simulink model "Cascaded_H_Bridge_Inverter"  (R2017a)
settings: Solver=VariableStepAuto  StartTime=0.0  StopTime=20e-3  MaxStep=1e-4  RelTol=1e-3
values from neighbouring files (symbols this model uses):
  Fs = 10000    [sequence_generator.m]
  o11 = zeros(1, Fs)    [sequence_generator.m]
  o13 = zeros(1, Fs)    [sequence_generator.m]
  o21 = zeros(1, Fs)    [sequence_generator.m]
  o23 = zeros(1, Fs)    [sequence_generator.m]
  p = 20e-3    (= 0.02)    [sequence_generator.m]
libraries: powerlib_meascontrol x37, powerlib x26, simulink x8
settings Model: Creator=Abubakar  LastModifiedBy=Abubakar

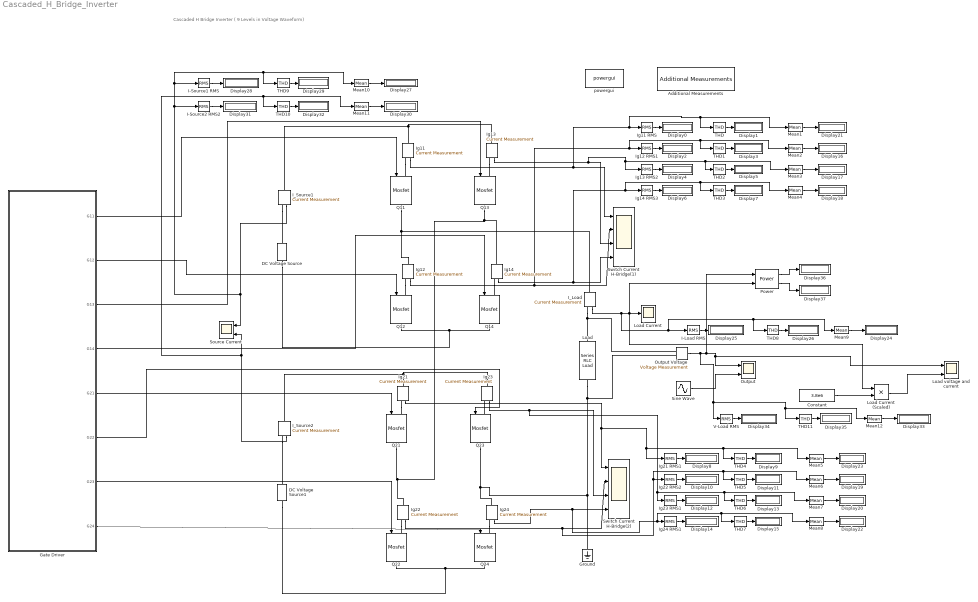
== system Cascaded_H_Bridge_Inverter ==
  note: Cascaded H Bridge Inverter
      | ( 9 Levels in Voltage Waveform)
  Additional Measurements : powerlib/Measurements/Additional Measurements  SystemSampleTime=-1
      settings: SourceProductName=Simscape Power Systems  SourceProductBaseCode=PS
  Constant : Constant  Value=3.8e6
  DC Voltage Source : powerlib/Electrical Sources/DC Voltage Source  Amplitude=10000  Measurements=None
  DC Voltage Source1 : powerlib/Electrical Sources/DC Voltage Source  Amplitude=30000  Measurements=None
  Display{0..37} (38 alike) : Display
  Gate Driver : Subsystem
  Ground : powerlib/Elements/Ground  LConnTagsString=a
  I-Load RMS : powerlib_meascontrol/Measurements/RMS  TrueRMS=on  Freq=50  RMSInit=0  Ts=0
  I-Source1 RMS : powerlib_meascontrol/Measurements/RMS  TrueRMS=on  Freq=50  RMSInit=0  Ts=0
  I-Source2 RMS2 : powerlib_meascontrol/Measurements/RMS  TrueRMS=on  Freq=50  RMSInit=0  Ts=0
  I_Load : powerlib/Measurements/Current Measurement  PhasorSimulation=off  OutputType=Complex  PSBequivalent=0
  I_Source1 : powerlib/Measurements/Current Measurement  PhasorSimulation=off  OutputType=Complex  PSBequivalent=0
  I_Source2 : powerlib/Measurements/Current Measurement  PhasorSimulation=off  OutputType=Complex  PSBequivalent=0
  Ig{11..14,21..24} (8 alike) : powerlib/Measurements/Current Measurement  PhasorSimulation=off  OutputType=Complex  PSBequivalent=0
  Ig11 RMS : powerlib_meascontrol/Measurements/RMS  TrueRMS=on  Freq=50  RMSInit=0  Ts=0
  Ig12 RMS1 : powerlib_meascontrol/Measurements/RMS  TrueRMS=on  Freq=50  RMSInit=0  Ts=0
  Ig13 RMS2 : powerlib_meascontrol/Measurements/RMS  TrueRMS=on  Freq=50  RMSInit=0  Ts=0
  Ig14 RMS3 : powerlib_meascontrol/Measurements/RMS  TrueRMS=on  Freq=50  RMSInit=0  Ts=0
  Ig21 RMS1 : powerlib_meascontrol/Measurements/RMS  TrueRMS=on  Freq=50  RMSInit=0  Ts=0
  Ig22 RMS2 : powerlib_meascontrol/Measurements/RMS  TrueRMS=on  Freq=50  RMSInit=0  Ts=0
  Ig23 RMS1 : powerlib_meascontrol/Measurements/RMS  TrueRMS=on  Freq=50  RMSInit=0  Ts=0
  Ig24 RMS1 : powerlib_meascontrol/Measurements/RMS  TrueRMS=on  Freq=50  RMSInit=0  Ts=0
  Load : powerlib/Elements/Series RLC Load  LConnTagsString=a  RConnTagsString=__new0  NominalVoltage=2.5e4  NominalFrequency=50  ActivePower=100  InductivePower=0  CapacitivePower=0  Setx0=off  InitialVoltage=0  SetiL0=off  InitialCurrent=0  Measurements=None  LoadType=constant PQ
  Load Current : Scope
  Load Current (Scaled) : Product
  Load voltage and current : Scope  NumInputPorts=2
  Mean{1..12} (12 alike) : powerlib_meascontrol/Measurements/Mean  Freq=60  Vinit=0  Ts=0
  Output : Scope  NumInputPorts=2
  Output Voltage : powerlib/Measurements/Voltage Measurement  PhasorSimulation=off  OutputType=Complex  PSBequivalent=0
  Power : powerlib_meascontrol/Measurements/Power  Freq=50  Vinit=[1, 0]  Iinit=[1, 0]  Ts=0
      settings: SourceProductName=Simscape Power Systems
  Q{11..14,21..24} (8 alike) : powerlib/Power Electronics/Mosfet  Ron=0.0001  Lon=0  Rd=0.0001  Vfd=0  IC=0  Rs=1e5  Cs=inf  Measurements=off
  Sine Wave : Sin  Amplitude=40000  Frequency=2*pi*(1/p)  SampleTime=0
  Source Current : Scope  NumInputPorts=2
  Switch Current H-Bridge(1) : Scope  NumInputPorts=4
  Switch Current H-Bridge(2) : Scope  NumInputPorts=4
  THD{,1..11} (12 alike) : powerlib_meascontrol/Measurements/THD  Freq=50  Ts=0
  V-Load RMS : powerlib_meascontrol/Measurements/RMS  TrueRMS=on  Freq=50  RMSInit=0  Ts=0
  powergui : powerlib/powergui  Priority=1  SimulationMode=Continuous  SampleTime=50e-6  frequency=60  Iterations=50  frequencyindice=0  Pbase=100e6  ErrMax=1e-4  UnitsV=kV  UnitsW=MW  buscounter=0  FunctionMessages=off  echomessages=off  EnableUseOfTLC=off  CurrentSourceSwitches=off  DisableSnubberDevices=off  DisableRonSwitches=off  DisableVfSwitches=off  DisplayEquations=off  SolverType=Tustin/Backward Euler (TBE)  Interpol=off  ExternalGateDelay=off  methode=off  Ts=100  x0status=blocks  SPID=on  SwTol=0  HookPort=off  RestoreLinks=warning  ResistiveCurrentMeasurement=off  Frange=[0:2:500]  Ylog=off  Xlog=on  ShowGrid=off  save=off  variable=ZData  structure=OutputData  ZoomFFT=off  StartTime=0  cycles=2  DisplayStyle=1  fundamental=50  FreqAxis=on  MaxFrequency=1000  frequencyindicesteady=1  RmsSteady=1  display=off
  wires:
  Gate Driver/1(G11) -> Q11/1
  Gate Driver/2(G12) -> Q12/1
  Gate Driver/3(G13) -> Q13/1
  Gate Driver/4(G14) -> Q14/1
  Gate Driver/5(G21) -> Q21/1
  Gate Driver/6(G22) -> Q23/1
  Gate Driver/7(G23) -> Q22/1
  Gate Driver/8(G24) -> Q24/1
  Sine Wave/1 -> Output/2
  Ig11/1 -> Mean1/1, THD/1, Ig11 RMS/1, Switch Current H-Bridge(1)/1
  Ig12/1 -> Mean2/1, THD1/1, Ig12 RMS1/1, Switch Current H-Bridge(1)/2
  Ig13/1 -> Mean3/1, THD2/1, Ig13 RMS2/1, Switch Current H-Bridge(1)/3
  Ig14/1 -> Mean4/1, THD3/1, Ig14 RMS3/1, Switch Current H-Bridge(1)/4
  Ig21/1 -> Mean5/1, THD4/1, Ig21 RMS1/1, Switch Current H-Bridge(2)/1
  Ig22/1 -> Mean6/1, THD5/1, Ig22 RMS2/1, Switch Current H-Bridge(2)/2
  Ig23/1 -> Mean7/1, THD6/1, Ig23 RMS1/1, Switch Current H-Bridge(2)/3
  Ig24/1 -> Mean8/1, THD7/1, Ig24 RMS1/1, Switch Current H-Bridge(2)/4
  THD/1 -> Display1/1
  Ig11 RMS/1 -> Display0/1
  Ig12 RMS1/1 -> Display2/1
  THD1/1 -> Display3/1
  THD2/1 -> Display5/1
  Ig13 RMS2/1 -> Display4/1
  Ig14 RMS3/1 -> Display6/1
  THD3/1 -> Display7/1
  THD7/1 -> Display15/1
  Ig24 RMS1/1 -> Display14/1
  Ig23 RMS1/1 -> Display12/1
  THD6/1 -> Display13/1
  THD5/1 -> Display11/1
  Ig22 RMS2/1 -> Display10/1
  Ig21 RMS1/1 -> Display8/1
  THD4/1 -> Display9/1
  Mean1/1 -> Display21/1
  Mean2/1 -> Display16/1
  Mean3/1 -> Display17/1
  Mean4/1 -> Display18/1
  Mean8/1 -> Display22/1
  Mean7/1 -> Display20/1
  Mean6/1 -> Display19/1
  Mean5/1 -> Display23/1
  Mean9/1 -> Display24/1
  THD8/1 -> Display26/1
  I-Load RMS/1 -> Display25/1
  I_Load/1 -> Mean9/1, THD8/1, I-Load RMS/1, Load Current (Scaled)/1, Power/2, Load Current/1
  I_Source1/1 -> I-Source2 RMS2/1, I-Source1 RMS/1, THD9/1, Mean10/1, Source Current/1
  I-Source1 RMS/1 -> Display28/1
  THD9/1 -> Display29/1
  Mean10/1 -> Display27/1
  Mean11/1 -> Display30/1
  THD10/1 -> Display32/1
  I-Source2 RMS2/1 -> Display31/1
  I_Source2/1 -> Mean11/1, THD10/1, Source Current/2
  Output Voltage/1 -> THD11/1, Mean12/1, V-Load RMS/1, Power/1, Load voltage and current/1, Output/1
  V-Load RMS/1 -> Display34/1
  THD11/1 -> Display35/1
  Mean12/1 -> Display33/1
  Power/1 -> Display36/1
  Power/2 -> Display37/1
  Load Current (Scaled)/1 -> Load voltage and current/2
  Constant/1 -> Load Current (Scaled)/2
  connections:
  Ig13/LConn1 -- I_Source1/LConn1 -- Ig11/LConn1
  Q11/RConn1 -- I_Load/LConn1 -- Ig12/LConn1
  Q12/RConn1 -- DC Voltage Source/LConn1 -- Q14/RConn1
  Ig21/LConn1 -- I_Source2/LConn1 -- Ig23/LConn1
  Q22/RConn1 -- DC Voltage Source1/LConn1 -- Q24/RConn1
  Q13/RConn1 -- Ig22/LConn1 -- Q21/RConn1 -- Ig14/LConn1
  Q23/RConn1 -- Ig24/LConn1 -- Load/RConn1 -- Output Voltage/LConn2 -- Ground/LConn1
  Ig11/RConn1 -- Q11/LConn1
  Ig13/RConn1 -- Q13/LConn1
  Ig12/RConn1 -- Q12/LConn1
  Ig14/RConn1 -- Q14/LConn1
  Ig23/RConn1 -- Q23/LConn1
  Ig21/RConn1 -- Q21/LConn1
  Ig24/RConn1 -- Q24/LConn1
  Ig22/RConn1 -- Q22/LConn1
  Output Voltage/LConn1 -- I_Load/RConn1 -- Load/LConn1
  I_Source1/RConn1 -- DC Voltage Source/RConn1
  I_Source2/RConn1 -- DC Voltage Source1/RConn1

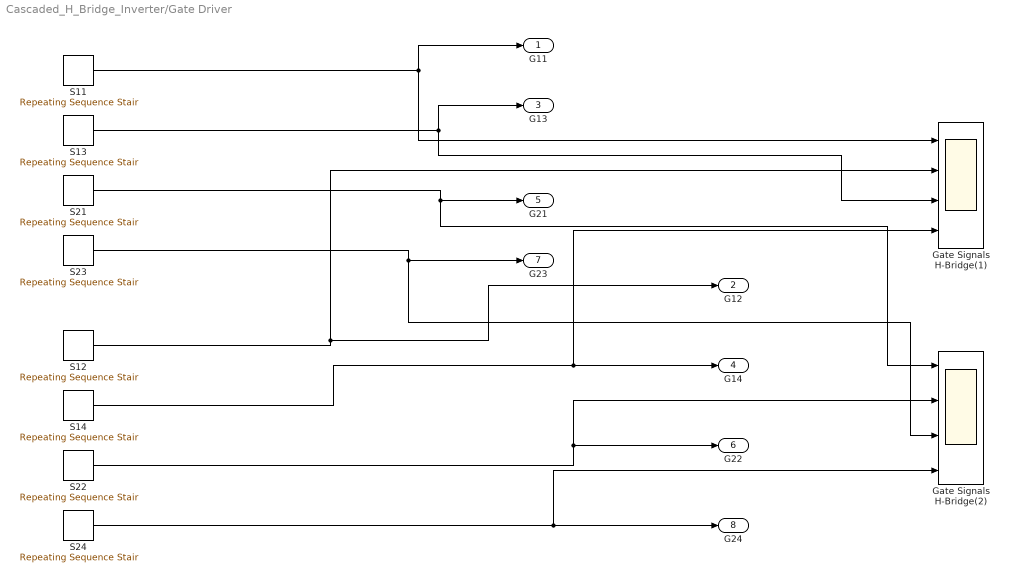
== system Cascaded_H_Bridge_Inverter/Gate Driver ==
  Gate Signals H-Bridge(1) : Scope  NumInputPorts=4
  Gate Signals H-Bridge(2) : Scope  NumInputPorts=4
  S11 : simulink/Sources/Repeating Sequence Stair  OutValues=o11'  tsamp=(p/Fs)  OutMin=[]  OutMax=[]  OutDataTypeStr=double  OutputDataTypeScalingMode=double  OutDataType=fixdt(0,8)  ConRadixGroup=Best Precision: Vector-wise  OutScaling=2^-12
  S12 : simulink/Sources/Repeating Sequence Stair  OutValues=~o11'  tsamp=(p/Fs)  OutMin=[]  OutMax=[]  OutDataTypeStr=double  OutputDataTypeScalingMode=double  OutDataType=fixdt(0,8)  ConRadixGroup=Best Precision: Vector-wise  OutScaling=2^-12
  S13 : simulink/Sources/Repeating Sequence Stair  OutValues=o13'  tsamp=(p/Fs)  OutMin=[]  OutMax=[]  OutDataTypeStr=double  OutputDataTypeScalingMode=double  OutDataType=fixdt(0,8)  ConRadixGroup=Best Precision: Vector-wise  OutScaling=2^-12
  S14 : simulink/Sources/Repeating Sequence Stair  OutValues=~o13'  tsamp=(p/Fs)  OutMin=[]  OutMax=[]  OutDataTypeStr=double  OutputDataTypeScalingMode=double  OutDataType=fixdt(0,8)  ConRadixGroup=Best Precision: Vector-wise  OutScaling=2^-12
  S21 : simulink/Sources/Repeating Sequence Stair  OutValues=o21'  tsamp=(p/Fs)  OutMin=[]  OutMax=[]  OutDataTypeStr=double  OutputDataTypeScalingMode=double  OutDataType=fixdt(0,8)  ConRadixGroup=Best Precision: Vector-wise  OutScaling=2^-12
  S22 : simulink/Sources/Repeating Sequence Stair  OutValues=~o21'  tsamp=(p/Fs)  OutMin=[]  OutMax=[]  OutDataTypeStr=double  OutputDataTypeScalingMode=double  OutDataType=fixdt(0,8)  ConRadixGroup=Best Precision: Vector-wise  OutScaling=2^-12
  S23 : simulink/Sources/Repeating Sequence Stair  OutValues=o23'  tsamp=(p/Fs)  OutMin=[]  OutMax=[]  OutDataTypeStr=double  OutputDataTypeScalingMode=double  OutDataType=fixdt(0,8)  ConRadixGroup=Best Precision: Vector-wise  OutScaling=2^-12
  S24 : simulink/Sources/Repeating Sequence Stair  OutValues=~o23'  tsamp=(p/Fs)  OutMin=[]  OutMax=[]  OutDataTypeStr=double  OutputDataTypeScalingMode=double  OutDataType=fixdt(0,8)  ConRadixGroup=Best Precision: Vector-wise  OutScaling=2^-12
  G11 : Outport
  G12 : Outport  Port=2
  G13 : Outport  Port=3
  G14 : Outport  Port=4
  G21 : Outport  Port=5
  G22 : Outport  Port=6
  G23 : Outport  Port=7
  G24 : Outport  Port=8
  wires:
  S11/1 -> G11/1, Gate Signals H-Bridge(1)/1
  S13/1 -> G13/1, Gate Signals H-Bridge(1)/3
  S21/1 -> Gate Signals H-Bridge(2)/1, G21/1
  S23/1 -> Gate Signals H-Bridge(2)/3, G23/1
  S12/1 -> Gate Signals H-Bridge(1)/2, G12/1
  S14/1 -> Gate Signals H-Bridge(1)/4, G14/1
  S22/1 -> Gate Signals H-Bridge(2)/2, G22/1
  S24/1 -> Gate Signals H-Bridge(2)/4, G24/1
